simulink model "nid_cvst_depth"  (Simulink 10.0)
settings: Solver=FixedStepDiscrete  StartTime=0.0  StopTime=inf  RelTol=1e-3  EnableMultiTasking=on
libraries: vipsnks x2, nid_lib x2
settings Model: Creator=tchikama  LastModifiedBy=bhisma
settings DataIOCC: LimitDataPoints=on  SignalLoggingSaveFormat=ModelDataLogs  SaveOutput=off
settings OptimizationCC: ExpressionDepthLimit=2147483647  SimCompilerOptimization=on
settings DebuggingCC: SolverPrmCheckMsg=warning  FcnCallInpInsideContextMsg=warning  StateNameClashWarn=warning
settings HardwareCC: ProdIntDivRoundTo=Zero  ProdEndianess=LittleEndian  ProdHWDeviceType=Generic->32-bit x86 compatible
settings RTWCC: RTWCompilerOptimization=on
settings CodeAppCC: MaxIdLength=95
settings GRTTargetCC: GeneratePreprocessorConditionals=Disable all
settings ConfigComp: CovExternalEMLEnable=off

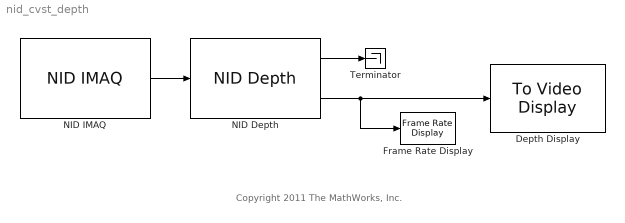
== system nid_cvst_depth ==
  note: Copyright 2011 The MathWorks, Inc.
  Depth Display : vipsnks/To Video Display  inputType=Obsolete  imagePorts=One multidimensional signal  OutputDevice=On-screen video monitor  fullScreen=off  videoWindowX=872  videoWindowY=185  saveWindowSize=off  videoWindowWidth=640  videoWindowHeight=480  dataOrg=Column-major  openAtMdlStart=on  isWindowOpen=on
      settings: SourceProductName=Computer Vision Toolbox  SourceProductBaseCode=VP
  Frame Rate Display : vipsnks/Frame Rate Display  UpdateRate=10
      settings: SourceProductName=Computer Vision Toolbox  SourceProductBaseCode=VP
  NID Depth : nid_lib/NID Depth  depthOutput=Depth  conv_XYZ_RW=off  viewer=on
  NID IMAQ : nid_lib/NID IMAQ  imaq_depth=on  imaq_motion=off  imaq_image=off  view_point=off  imaq_skeleton=off  imaq_ir=off  mirror_image=off  imaq_sample_time=1/30  res_fps=VGA (640x480): 30 FPS  angle=0  angle_read=off  near_mode=off
  Terminator : Terminator
  wires:
  NID IMAQ/1 -> NID Depth/1
  NID Depth/2 -> Depth Display/1, Frame Rate Display/1
  NID Depth/1 -> Terminator/1
